simulink model "RC_EVAP"  (Simulink 9.2)
settings: Solver=ode1  StartTime=0.0  StopTime=30000  FixedStep=0.1  RelTol=1e-3  EnableMultiTasking=on
settings Model: Creator=Natalia  LastModifiedBy=user
settings OptimizationCC: ExpressionDepthLimit=2147483647
settings DebuggingCC: SolverPrmCheckMsg=warning
settings ConfigComp: CovHTMLOptions=-aTS=1 -bRG=1 -bTC=1 -hTR=0 -nFC=0 -scm=1 -bcm=1 -xEv=0  CovSFcnEnable=off

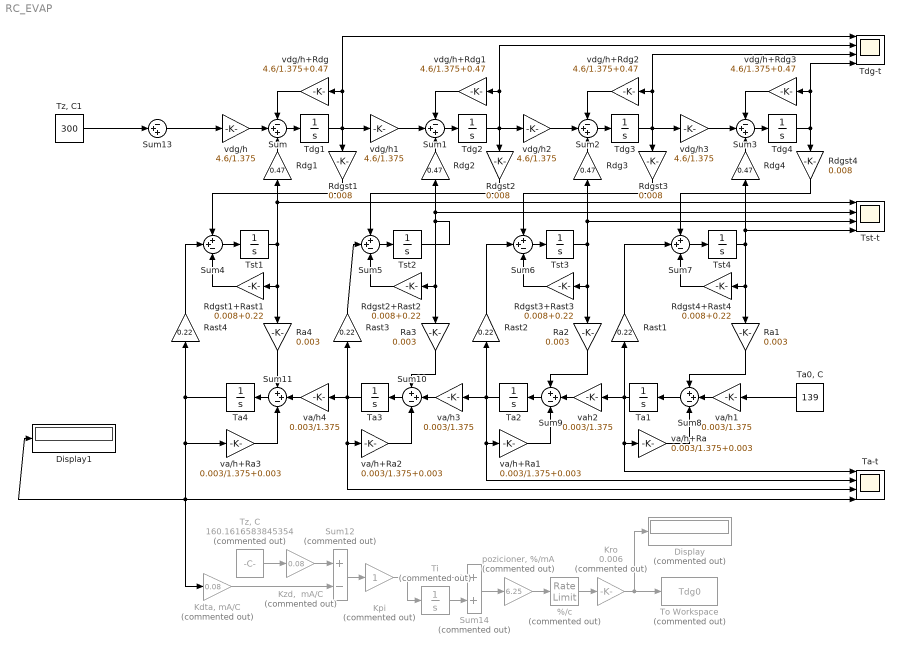
== system RC_EVAP ==
  %/c : RateLimiter  Commented=on  RisingSlewLimit=5  FallingSlewLimit=-5  SampleTimeMode=inherited
  Display : Display  Commented=on
  Display1 : Display
  "Kdta, mA/C" : Gain  Commented=on  Gain=0.08
  Kpi : Gain  Commented=on
  Kro : Gain  Commented=on  Gain=0.006
  "Kzd,  mA/C" : Gain  Commented=on  Gain=0.08
  Ra{1..4} (4 alike) : Gain  Gain=0.003
  Rast{1..4} (4 alike) : Gain  Gain=0.22
  Rdg{1..4} (4 alike) : Gain  Gain=0.47
  Rdgst{1..4} (4 alike) : Gain  Gain=0.008
  Rdgst1+Rast1 : Gain  Gain=0.008+0.22
  Rdgst2+Rast2 : Gain  Gain=0.008+0.22
  Rdgst3+Rast3 : Gain  Gain=0.008+0.22
  Rdgst4+Rast4 : Gain  Gain=0.008+0.22
  Sum{,1..3,13} (5 alike) : Sum  Inputs=-++
  Sum{4..11} (8 alike) : Sum  Inputs=++-
  Sum12 : Sum  Commented=on  Inputs=+-
  Sum14 : Sum  Commented=on
  Ta-t : Scope  NumInputPorts=4
  "Ta0, C" : Constant  Value=139
  Ta1 : Integrator  InitialCondition=143.67340
  Ta2 : Integrator  InitialCondition=148.736080
  Ta3 : Integrator  InitialCondition=154.220450
  Ta4 : Integrator  InitialCondition=160.161650
  Tdg-t : Scope  NumInputPorts=4
  Tdg1 : Integrator  InitialCondition=283.30650
  Tdg2 : Integrator  InitialCondition=267.89660
  Tdg3 : Integrator  InitialCondition=253.67150
  Tdg4 : Integrator  InitialCondition=240.54030
  Ti : Integrator  Commented=on  InitialCondition=8000  UpperSaturationLimit=8012  LowerSaturationLimit=6012
  To Workspace : ToWorkspace  Commented=on  VariableName=Tdg0  SampleTime=-1
  Tst-t : Scope  NumInputPorts=4
  Tst1 : Integrator  InitialCondition=164.48250
  Tst2 : Integrator  InitialCondition=158.20900
  Tst3 : Integrator  InitialCondition=152.41800
  Tst4 : Integrator  InitialCondition=147.07220
  "Tz, C" : Constant  Commented=on  Value=160.1616583845354
  "Tz, C1" : Constant  Value=300
  "pozicioner, %/mA" : Gain  Commented=on  Gain=6.25
  va/h+Ra{,1..3} (4 alike) : Gain  Gain=0.003/1.375+0.003
  va/h1 : Gain  Gain=0.003/1.375
  va/h3 : Gain  Gain=0.003/1.375
  va/h4 : Gain  Gain=0.003/1.375
  vah2 : Gain  Gain=0.003/1.375
  vdg/h{,1..3} (4 alike) : Gain  Gain=4.6/1.375
  vdg/h+Rdg{,1..3} (4 alike) : Gain  Gain=4.6/1.375+0.47
  wires:
  vdg/h/1 -> Sum/2
  vdg/h+Rdg/1 -> Sum/1
  Sum/1 -> Tdg1/1
  Tdg1/1 -> vdg/h+Rdg/1, Tdg-t/1, vdg/h1/1, Rdgst1/1
  vdg/h1/1 -> Sum1/2
  vdg/h+Rdg1/1 -> Sum1/1
  Sum1/1 -> Tdg2/1
  Tdg2/1 -> vdg/h+Rdg1/1, Tdg-t/2, Rdgst2/1, vdg/h2/1
  vdg/h2/1 -> Sum2/2
  vdg/h+Rdg2/1 -> Sum2/1
  Sum2/1 -> Tdg3/1
  Tdg3/1 -> vdg/h+Rdg2/1, Tdg-t/3, vdg/h3/1, Rdgst3/1
  vdg/h3/1 -> Sum3/2
  vdg/h+Rdg3/1 -> Sum3/1
  Sum3/1 -> Tdg4/1
  Tdg4/1 -> vdg/h+Rdg3/1, Tdg-t/4, Rdgst4/1
  Rdg1/1 -> Sum/3
  Rdg2/1 -> Sum1/3
  Rdg3/1 -> Sum2/3
  Rdg4/1 -> Sum3/3
  Sum4/1 -> Tst1/1
  Sum5/1 -> Tst2/1
  Sum6/1 -> Tst3/1
  Sum7/1 -> Tst4/1
  Tst4/1 -> Rdgst4+Rast4/1, Ra1/1, Rdg4/1, Tst-t/4
  Rdgst4+Rast4/1 -> Sum7/3
  Tst3/1 -> Rdgst3+Rast3/1, Ra2/1, Rdg3/1, Tst-t/3
  Rdgst3+Rast3/1 -> Sum6/3
  Tst2/1 -> Rdg2/1, Tst-t/2, Rdgst2+Rast2/1, Ra3/1
  Tst1/1 -> Rdgst1+Rast1/1, Ra4/1, Rdg1/1, Tst-t/1
  Rdgst1+Rast1/1 -> Sum4/3
  Rdgst1/1 -> Sum4/1
  Rdgst2/1 -> Sum5/1
  Rdgst3/1 -> Sum6/1
  Rdgst4/1 -> Sum7/1
  Rdgst2+Rast2/1 -> Sum5/3
  va/h1/1 -> Sum8/2
  va/h+Ra/1 -> Sum8/3
  Ta1/1 -> Ta-t/1, va/h+Ra/1, Rast1/1, vah2/1
  vah2/1 -> Sum9/2
  va/h+Ra1/1 -> Sum9/3
  Sum9/1 -> Ta2/1
  Ta2/1 -> va/h+Ra1/1, Ta-t/2, va/h3/1, Rast2/1
  va/h3/1 -> Sum10/2
  va/h+Ra2/1 -> Sum10/3
  Sum10/1 -> Ta3/1
  Ta3/1 -> va/h+Ra2/1, Ta-t/3, va/h4/1, Rast3/1
  va/h4/1 -> Sum11/2
  va/h+Ra3/1 -> Sum11/3
  Sum11/1 -> Ta4/1
  Ta4/1 -> "Kdta, mA/C"/1, Display1/1, Ta-t/4, va/h+Ra3/1, Rast4/1
  Rast4/1 -> Sum4/2
  Ra4/1 -> Sum11/1
  Rast3/1 -> Sum5/2
  Ra3/1 -> Sum10/1
  Rast2/1 -> Sum6/2
  Ra2/1 -> Sum9/1
  Rast1/1 -> Sum7/2
  Ra1/1 -> Sum8/1
  "Tz, C"/1 -> "Kzd,  mA/C"/1
  "Kdta, mA/C"/1 -> Sum12/2
  "Kzd,  mA/C"/1 -> Sum12/1
  Kro/1 -> To Workspace/1, Display/1
  "pozicioner, %/mA"/1 -> %/c/1
  %/c/1 -> Kro/1
  Sum14/1 -> "pozicioner, %/mA"/1
  Sum12/1 -> Kpi/1
  Ti/1 -> Sum14/2
  Kpi/1 -> Sum14/1, Ti/1
  "Ta0, C"/1 -> va/h1/1
  Sum13/1 -> vdg/h/1
  "Tz, C1"/1 -> Sum13/2
  Sum8/1 -> Ta1/1
